simulink library "dspmrf_lib"  (Simulink 3.00)
PreLoadFcn:
  | load dspmrf_coeffs
undefined symbols (not defined in the file or in its folder): mrf_firdn1, mrf_upfir1
libraries: dspmlti3 x16, dspmrf_lib x4
settings Model: Creator=don  LastModifiedBy=don

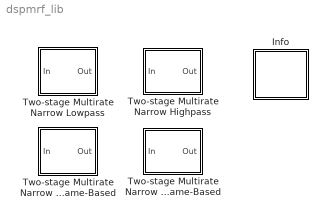
== system dspmrf_lib ==
  Info : Subsystem
      mask Display: disp('Filters')
  Two-stage Multirate Narrow Highpass : Subsystem
  Two-stage Multirate Narrow Highpass Frame-Based : Subsystem
  Two-stage Multirate Narrow Lowpass : Subsystem
  Two-stage Multirate Narrow Lowpass Frame-Based : Subsystem

== system dspmrf_lib/Info ==
  note: To design the filters used in the underlying blocks:
      |
      | mrf_firdn1 = remez(684,[0 .0733 .0833 1],[1 1 0 0],[1 50]);
      | mrf_firdn2 = remez(451,[0 .225 .24 1],[1 1 0 0],[1 50]);
      |
      | mrf_upfir2 = remez(451,[0 .225 .24 1],[1 1 0 0],[1 50]) * 4;
      | mrf_upfir1 = remez(684,[0 .0733 .0833 1],[1 1 0 0],[1 50]) * 12;

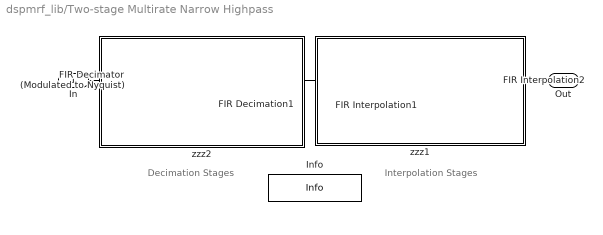
== system dspmrf_lib/Two-stage Multirate Narrow Highpass ==
  note: Decimation Stages
  note: Interpolation Stages
  In : Inport  Port=1
  FIR Decimation1 : dspmlti3/FIR Decimation  h=mrf_firdn2  D=4  framing=Maintain input frame size
  FIR Interpolation1 : dspmlti3/FIR Interpolation  h=mrf_upfir2  L=4  framing=Maintain input frame size
  FIR Interpolation2 : dspmlti3/FIR Interpolation  h=mrf_upfir1 .* ((-1).^(0:684))  L=12  framing=Maintain input frame size
  FIR Decimator (Modulated to Nyquist) : dspmlti3/FIR Decimation  h=mrf_firdn1 .* ((-1).^(0:684))  D=12  framing=Maintain input frame size
  Info : dspmrf_lib/Info
  zzz1 : Subsystem
      settings: OpenFcn=dspmsmrff;
      mask Display: disp('')
  zzz2 : Subsystem
      settings: OpenFcn=dspmsmrff;
      mask Display: disp('')
  Out : Outport  Port=1
  wires:
  In/1 -> FIR Decimator (Modulated to Nyquist)/1
  FIR Decimator (Modulated to Nyquist)/1 -> FIR Decimation1/1
  FIR Decimation1/1 -> FIR Interpolation1/1
  FIR Interpolation1/1 -> FIR Interpolation2/1
  FIR Interpolation2/1 -> Out/1

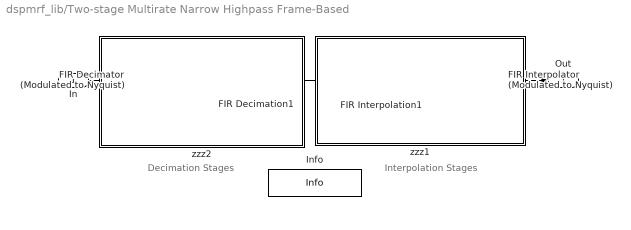
== system dspmrf_lib/Two-stage Multirate Narrow Highpass Frame-Based ==
  note: Interpolation Stages
  note: Decimation Stages
  In : Inport  Port=1
  FIR Decimation1 : dspmlti3/FIR Decimation  h=mrf_firdn2  D=4  framing=Maintain input frame rate
  FIR Interpolation1 : dspmlti3/FIR Interpolation  h=mrf_upfir2  L=4  framing=Maintain input frame rate
  FIR Decimator (Modulated to Nyquist) : dspmlti3/FIR Decimation  h=mrf_firdn1 .* ((-1).^(0:684))  D=12  framing=Maintain input frame rate
  FIR Interpolator (Modulated to Nyquist) : dspmlti3/FIR Interpolation  h=mrf_upfir1 .* ((-1).^(0:684))  L=12  framing=Maintain input frame rate
  Info : dspmrf_lib/Info
  zzz1 : Subsystem
      settings: OpenFcn=dspmsmrff;
      mask Display: disp('')
  zzz2 : Subsystem
      settings: OpenFcn=dspmsmrff;
      mask Display: disp('')
  Out : Outport  Port=1
  wires:
  FIR Interpolator (Modulated to Nyquist)/1 -> Out/1
  FIR Interpolation1/1 -> FIR Interpolator (Modulated to Nyquist)/1
  FIR Decimation1/1 -> FIR Interpolation1/1
  FIR Decimator (Modulated to Nyquist)/1 -> FIR Decimation1/1
  In/1 -> FIR Decimator (Modulated to Nyquist)/1

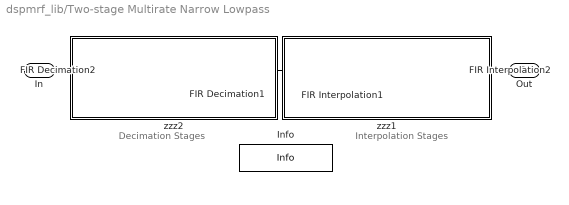
== system dspmrf_lib/Two-stage Multirate Narrow Lowpass ==
  note: Decimation Stages
  note: Interpolation Stages
  In : Inport  Port=1
  FIR Decimation1 : dspmlti3/FIR Decimation  h=mrf_firdn2  D=4  framing=Maintain input frame size
  FIR Decimation2 : dspmlti3/FIR Decimation  h=mrf_firdn1  D=12  framing=Maintain input frame size
  FIR Interpolation1 : dspmlti3/FIR Interpolation  h=mrf_upfir2  L=4  framing=Maintain input frame size
  FIR Interpolation2 : dspmlti3/FIR Interpolation  h=mrf_upfir1  L=12  framing=Maintain input frame size
  Info : dspmrf_lib/Info
  zzz1 : Subsystem
      settings: OpenFcn=dspmsmrff;
      mask Display: disp('')
  zzz2 : Subsystem
      settings: OpenFcn=dspmsmrff;
      mask Display: disp('')
  Out : Outport  Port=1
  wires:
  In/1 -> FIR Decimation2/1
  FIR Decimation2/1 -> FIR Decimation1/1
  FIR Decimation1/1 -> FIR Interpolation1/1
  FIR Interpolation1/1 -> FIR Interpolation2/1
  FIR Interpolation2/1 -> Out/1

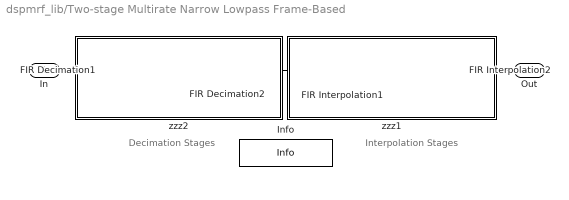
== system dspmrf_lib/Two-stage Multirate Narrow Lowpass Frame-Based ==
  note: Decimation Stages
  note: Interpolation Stages
  In : Inport  Port=1
  FIR Decimation1 : dspmlti3/FIR Decimation  h=mrf_firdn1  D=12  framing=Maintain input frame rate
  FIR Decimation2 : dspmlti3/FIR Decimation  h=mrf_firdn2  D=4  framing=Maintain input frame rate
  FIR Interpolation1 : dspmlti3/FIR Interpolation  h=mrf_upfir2  L=4  framing=Maintain input frame rate
  FIR Interpolation2 : dspmlti3/FIR Interpolation  h=mrf_upfir1  L=12  framing=Maintain input frame rate
  Info : dspmrf_lib/Info
  zzz1 : Subsystem
      settings: OpenFcn=dspmsmrff;
      mask Display: disp('')
  zzz2 : Subsystem
      settings: OpenFcn=dspmsmrff;
      mask Display: disp('')
  Out : Outport  Port=1
  wires:
  FIR Interpolation2/1 -> Out/1
  FIR Interpolation1/1 -> FIR Interpolation2/1
  FIR Decimation2/1 -> FIR Interpolation1/1
  FIR Decimation1/1 -> FIR Decimation2/1
  In/1 -> FIR Decimation1/1

== system dspmrf_lib/Two-stage Multirate Narrow Highpass/zzz1 ==

== system dspmrf_lib/Two-stage Multirate Narrow Highpass/zzz2 ==

== system dspmrf_lib/Two-stage Multirate Narrow Highpass Frame-Based/zzz1 ==

== system dspmrf_lib/Two-stage Multirate Narrow Highpass Frame-Based/zzz2 ==

== system dspmrf_lib/Two-stage Multirate Narrow Lowpass/zzz1 ==

== system dspmrf_lib/Two-stage Multirate Narrow Lowpass/zzz2 ==

== system dspmrf_lib/Two-stage Multirate Narrow Lowpass Frame-Based/zzz1 ==

== system dspmrf_lib/Two-stage Multirate Narrow Lowpass Frame-Based/zzz2 ==
